simulink model "lev_state"  (R2021b)
settings: Solver=VariableStepAuto  StartTime=0.0  StopTime=80.0  RelTol=1e-3
values from neighbouring files (symbols this model uses):
  a = i1^2*z1/((l^2+z1^2)^(3/2))    (= 959.854675025)    [MagLev4coils.m]
  b = i1^2*l/((l^2+z1^2)^(3/2))    (= 907.062667899)    [MagLev4coils.m]
  x0 = [-0.25;0;0;0;0]    [MagLev.m]
undefined symbols (not defined in the file or in its folder): c, d
settings Model: Creator=ik76  LastModifiedBy=ik76
settings SolverCC: ZeroCrossAlgorithm=Adaptive
settings OptimizationCC: BlockReduction=off  BooleanDataType=off
settings DebuggingCC: SaveWithParameterizedLinksMsg=none  UnderspecifiedInitializationDetection=Classic  MergeDetectMultiDrivingBlocksExec=none  SignalResolutionControl=TryResolveAllWithWarning  IgnoredZcDiagnostic=none
settings HardwareCC: TargetUnknown=on
settings ModelReferenceCC: PropagateSignalLabelsOutOfModel=off

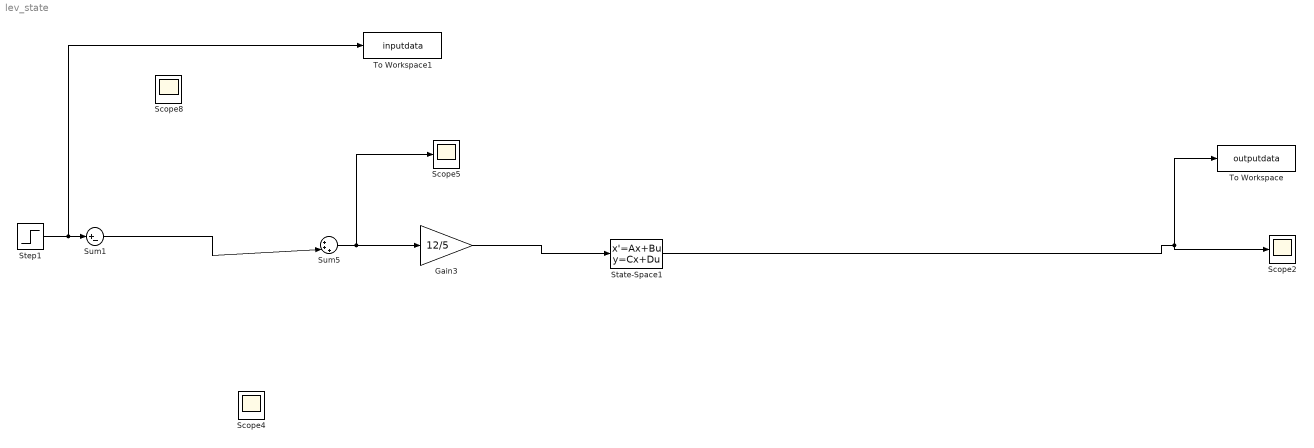
== system lev_state ==
  Gain3 : Gain  Gain=12/5
  Scope{2,4..5,8} (4 alike) : Scope
  State-Space1 : StateSpace  A=a  B=b  C=c  D=d  InitialCondition=x0
  Step1 : Step  Time=0  After=2.5  SampleTime=0
  Sum1 : Sum  Inputs=|+-
  Sum5 : Sum  Inputs=|+++
  To Workspace : ToWorkspace  VariableName=outputdata  SaveFormat=Structure With Time  SampleTime=-1
  To Workspace1 : ToWorkspace  VariableName=inputdata  SaveFormat=Structure With Time  SampleTime=-1
  wires:
  Step1/1 -> To Workspace1/1, Sum1/1
  Gain3/1 -> State-Space1/1
  Sum1/1 -> Sum5/2
  Sum5/1 -> Gain3/1, Scope5/1
  State-Space1/1 -> To Workspace/1, Scope2/1
